simulink model "Copy"  (R2022a)
settings: Solver=VariableStepAuto  StartTime=0.0  StopTime=72  RelTol=1e-6
model workspace (MAT data in the model file):
  ROBOT = SerialLink
  ROBOT.name = 'PLUMA'
  ROBOT.gravity = [0; 0; 9.81]
  ROBOT.base = SE3
  ROBOT.base.data = [1  0  0  0; 0  1  0  0; 0  0  1  0; 0  0  0  1]
  ROBOT.tool = SE3
  ROBOT.tool.data = [1  0  0  0; 0  1  0  0; 0  0  1  0; 0  0  0  1]
  ROBOT.fast = 0
  ROBOT.n = 2
  ROBOT.links(1) = Link
  ROBOT.links(1).theta = 0
  ROBOT.links(1).d = 0
  ROBOT.links(1).alpha = 0
  ROBOT.links(1).a = 0.1
  ROBOT.links(1).jointtype = 'R'
  ROBOT.links(1).mdh = 0
  ROBOT.links(1).offset = 0
  ROBOT.links(1).flip = 0
  ROBOT.links(1).r = [0 0 0]
  ROBOT.links(1).I = [0  0  0; 0  0  0; 0  0  0]
  ROBOT.links(1).B = 0
  ROBOT.links(1).Tc = [0 0]
  ROBOT.links(1).G = 0
  ROBOT.links(2) = Link
  ROBOT.links(2).theta = 0
  ROBOT.links(2).d = -0.007
  ROBOT.links(2).alpha = 0
  ROBOT.links(2).a = 0.1
  ROBOT.links(2).jointtype = 'R'
  ROBOT.links(2).mdh = 0
  ROBOT.links(2).offset = 0
  ROBOT.links(2).flip = 0
  ROBOT.links(2).r = [0 0 0]
  ROBOT.links(2).I = [0  0  0; 0  0  0; 0  0  0]
  ROBOT.links(2).B = 0
  ROBOT.links(2).Tc = [0 0]
  ROBOT.links(2).G = 0
  ROBOT.mdh = 0
values from neighbouring files (symbols this model uses):
  lc_1 = 0.1    [PlumaBotDynamic.m]    (also in PlumaID.m; matlab.mat)
  lc_2 = 0.1    [PlumaBotDynamic.m]    (also in PlumaID.m; matlab.mat)
  m_1 = 0.01    [PlumaBotDynamic.m]    (also in PlumaID.m = PARAM(1,1); matlab.mat)
  m_2 = 0.01    [PlumaBotDynamic.m]    (also in PlumaID.m = m_1; matlab.mat)
  ROBOT = SerialLink([L1 L2])    [PlumaID.m]
undefined symbols (not defined in the file or in its folder): PlannarForwardKinematics
settings Model: PacingRate=100  Creator=sergi  LastModifiedBy=sergi
settings DataIOCC: ExternalInput=qd1_Sim qd2_Sim Tau1_Sim Tau2_Sim  LoadExternalInput=on

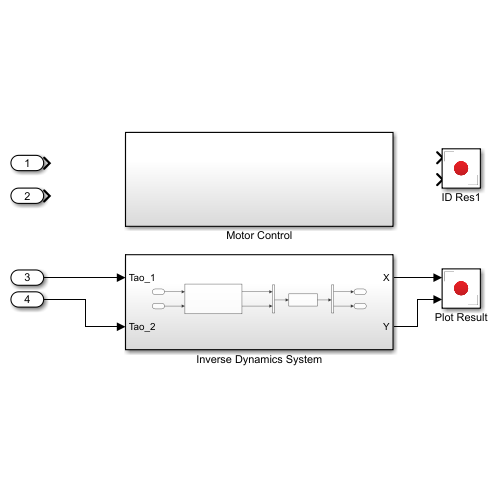
[thumbnail: Simulink's stored preview of the top-level diagram]
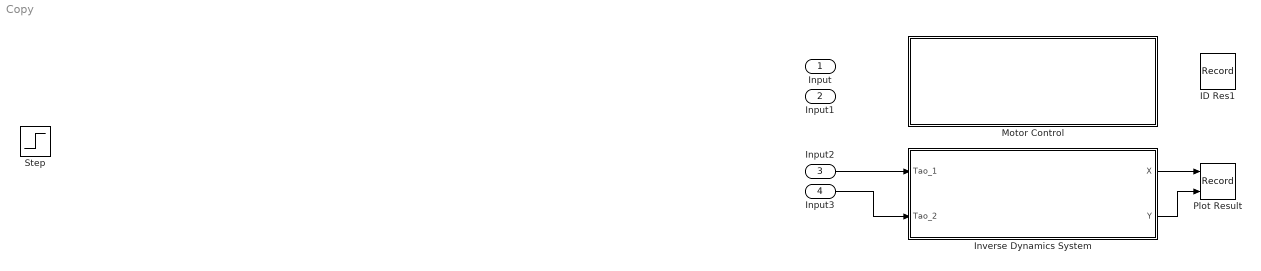
== system Copy ==
  Input : Inport
  Input1 : Inport  Port=2
  Input2 : Inport  Port=3
  Input3 : Inport  Port=4
  ID Res1 : Record  FileSettingsInternal="{\"entries\":[{\"content\":{\"excelSettings\":{\"content\":{},\"type\":\"Streamout.ExcelSettings\"}},\"type\":\"Streamout.FileSettingStorage\",\"uuid\":\"56932276-5bf3-452b-bf16-dfa087070347\"}],\"packageUris\":[\"http://schema.mathworks.com/mf0/streamout_blocks/R2020a\"],\"version\":\"1.0\"}"  Layout=[1 1]  SignalsInternal="{\"entries\":[{\"content\":{\"signals\":[{\"content\":{\"blockPath\":[\"Euler_Lagrange2DoF/ID Res1\"],\"channel\":[],\"dimensions\":[1],\"domain\":\"Euler_Lagrange2DoF/ID Res1\",\"lineColor\":\"#a2142f\",\"plots\":[1],\"port\":1,\"sid\":[],\"signalID\":3017,\"signalName\":\"Demux:1\"},\"type\":\"RecordBlkView.Signal\",\"uuid\":\"4088d432-ae20-42b7-817c-45be3513a391\"},{\"content\":{\"blockPath\":[\"Euler_Lagrange2DoF/ID Res1\"],\"channel\":[],\"dimensions\":[1],\"domain\":\"Euler_Lagrange2DoF/ID Res1\",\"lineColor\":\"#139fff\",\"plots\":[1],\"port\":2,\"sid\":[],\"signalID\":3020,\"signalName\":\"Demux:2\"},\"type\":\"RecordBlkView.Signal\",\"uuid\":\"2a97dab6-9d39-4673-b351-30ba74675ba8\"}]},\"type\":\"RecordBlkView.InputSignals\",\"uuid\":\"08b86e83-247f-44f9-93c2-be27e3250c02\"}],\"packageUris\":[\"http://schema.mathworks.com/mf0/streamout_blocks/R2020a\"],\"version\":\"1.0\"}"  VisualizationBindings="{\"xyplotplugin\":{\"info\":[{\"series\":[{\"bindingParametersList\":[{\"parameter\":\"X-Axis\",\"signalID\":3017,\"signalName\":\"Demux:1\"},{\"parameter\":\"Y-Axis\",\"signalID\":3020,\"signalName\":\"Demux:2\"}],\"seriesID\":58422}],\"subplotID\":1}]}}"  CompatibilityTag=XY
  Inverse Dynamics System : Subsystem
  Motor Control : Subsystem
  Plot Result : Record  FileSettingsInternal="{\"entries\":[{\"content\":{\"excelSettings\":{\"content\":{},\"type\":\"Streamout.ExcelSettings\"}},\"type\":\"Streamout.FileSettingStorage\",\"uuid\":\"fb85b01d-8259-4e48-a2a1-dabff8c76c20\"}],\"packageUris\":[\"http://schema.mathworks.com/mf0/streamout_blocks/R2020a\"],\"version\":\"1.0\"}"  Layout=[1 1]  SignalsInternal="{\"entries\":[{\"content\":{\"signals\":[{\"content\":{\"blockPath\":[\"Euler_Lagrange2DoF/Plot Result\"],\"channel\":[],\"dimensions\":[1],\"domain\":\"Euler_Lagrange2DoF/Plot Result\",\"lineColor\":\"#a2142f\",\"plots\":[1],\"port\":1,\"sid\":[],\"signalID\":3009,\"signalName\":\"Demux:1\"},\"type\":\"RecordBlkView.Signal\",\"uuid\":\"3bdfdfc0-49fd-4183-b95a-a6f0e32564c5\"},{\"content\":{\"blockPath\":[\"Euler_Lagrange2DoF/Plot Result\"],\"channel\":[],\"dimensions\":[1],\"domain\":\"Euler_Lagrange2DoF/Plot Result\",\"lineColor\":\"#139fff\",\"plots\":[1],\"port\":2,\"sid\":[],\"signalID\":3012,\"signalName\":\"Demux:2\"},\"type\":\"RecordBlkView.Signal\",\"uuid\":\"952c7ff3-3212-4a54-8455-608972501b81\"}]},\"type\":\"RecordBlkView.InputSignals\",\"uuid\":\"31803040-3250-4009-82ba-7b6bd40bd6b4\"}],\"packageUris\":[\"http://schema.mathworks.com/mf0/streamout_blocks/R2020a\"],\"version\":\"1.0\"}"  VisualizationBindings="{\"xyplotplugin\":{\"info\":[{\"series\":[{\"bindingParametersList\":[{\"parameter\":\"X-Axis\",\"signalID\":3009,\"signalName\":\"Demux:1\"},{\"parameter\":\"Y-Axis\",\"signalID\":3012,\"signalName\":\"Demux:2\"}],\"seriesID\":1739}],\"subplotID\":1}]}}"  CompatibilityTag=XY
  Step : Step  IOType=siggen  SampleTime=0
  wires:
  Inverse Dynamics System/1(X) -> Plot Result/1
  Inverse Dynamics System/2(Y) -> Plot Result/2
  Input2/1 -> Inverse Dynamics System/1(Tao_1)
  Input3/1 -> Inverse Dynamics System/2(Tao_2)

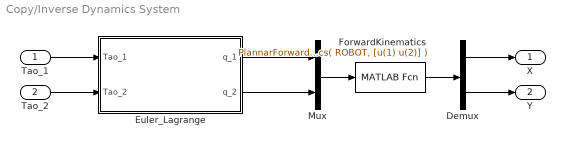
== system Copy/Inverse Dynamics System ==
  Tao_1 : Inport
  Tao_2 : Inport  Port=2
  Demux : Demux  Outputs=2
  Euler_Lagrange : Subsystem  TreatAsAtomicUnit=on
  ForwardKinematics : MATLABFcn  MATLABFcn=PlannarForwardKinematics( ROBOT, [u(1) u(2)] )  OutputDimensions=2
  Mux : Mux  Inputs=2
  X : Outport
  Y : Outport  Port=2
  wires:
  Euler_Lagrange/1(q_1) -> Mux/1
  ForwardKinematics/1 -> Demux/1
  Tao_2/1 -> Euler_Lagrange/2(Tao_2)
  Mux/1 -> ForwardKinematics/1
  Euler_Lagrange/2(q_2) -> Mux/2
  Demux/2 -> Y/1
  Demux/1 -> X/1
  Tao_1/1 -> Euler_Lagrange/1(Tao_1)

== system Copy/Motor Control ==

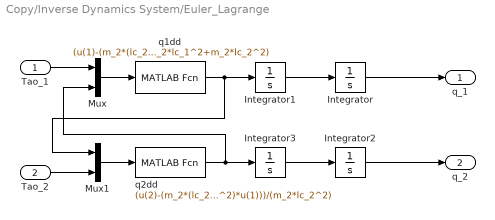
== system Copy/Inverse Dynamics System/Euler_Lagrange ==
  Tao_1 : Inport
  Tao_2 : Inport  Port=2
  Integrator{,1..3} (4 alike) : Integrator
  Mux : Mux  Inputs=2
  Mux1 : Mux  Inputs=2
  q1dd : MATLABFcn  MATLABFcn=(u(1)-(m_2*(lc_2^2)*u(2)))/(m_1*lc_1^2+m_2*lc_1^2+m_2*lc_2^2)
  q2dd : MATLABFcn  MATLABFcn=(u(2)-(m_2*(lc_2^2)*u(1)))/(m_2*lc_2^2)
  q_1 : Outport
  q_2 : Outport  Port=2
  wires:
  Mux/1 -> q1dd/1
  q2dd/1 -> Mux/2, Integrator3/1
  Tao_2/1 -> Mux1/2
  Mux1/1 -> q2dd/1
  q1dd/1 -> Mux1/1, Integrator1/1
  Integrator1/1 -> Integrator/1
  Integrator3/1 -> Integrator2/1
  Integrator/1 -> q_1/1
  Tao_1/1 -> Mux/1
  Integrator2/1 -> q_2/1
